simulink model "Optimal_reg_lqr"  (R2019a)
settings: Solver=VariableStepAuto  StartTime=0.0  StopTime=10.0  RelTol=1e-3
values from neighbouring files (symbols this model uses):
  A = [0 1 0 0;m*g*l(M+m)/d 0 0 m*l*b/d;0 0 0 1;-g*m^2*l^2/d 0 0 -b*(I+m*l^2)/d]    [inv_pend.m]
  B = [0;-m*l/d;0;(I+m*l^2)/d]    [inv_pend.m]
  C = [0 0 1 0;1 0 0 0]    [inv_pend.m]
  Kopt = lqr(A,B,Q,R)    [inv_pend.m]
  Vopt = 1/dcgain(ss(Ac,B,Cn,Dn))    [inv_pend.m]
settings Model: Creator=Naveen  LastModifiedBy=Naveen

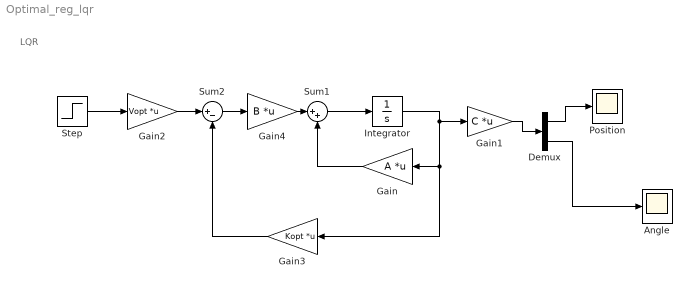
== system Optimal_reg_lqr ==
  note: LQR
  Angle : Scope
  Demux : Demux  Outputs=2
  Gain : Gain  Gain=A  Multiplication=Matrix(K*u)
  Gain1 : Gain  Gain=C  Multiplication=Matrix(K*u)
  Gain2 : Gain  Gain=Vopt  Multiplication=Matrix(K*u)
  Gain3 : Gain  Gain=Kopt  Multiplication=Matrix(K*u)
  Gain4 : Gain  Gain=B  Multiplication=Matrix(K*u)
  Integrator : Integrator
  Position : Scope
  Step : Step  Time=0  After=5  SampleTime=0
  Sum1 : Sum  Inputs=|++
  Sum2 : Sum  Inputs=|+-
  wires:
  Gain2/1 -> Sum2/1
  Gain/1 -> Sum1/2
  Gain1/1 -> Demux/1
  Gain3/1 -> Sum2/2
  Step/1 -> Gain2/1
  Demux/2 -> Angle/1
  Demux/1 -> Position/1
  Integrator/1 -> Gain1/1, Gain3/1, Gain/1
  Sum2/1 -> Gain4/1
  Sum1/1 -> Integrator/1
  Gain4/1 -> Sum1/1
